simulink model "powerwindow"  (Simulink 7.9)
settings: Solver=ode45  StartTime=0.0  StopTime=inf  RelTol=1e-3
libraries: simulink x3
settings Model: Creator=ia3803  LastModifiedBy=ia3803

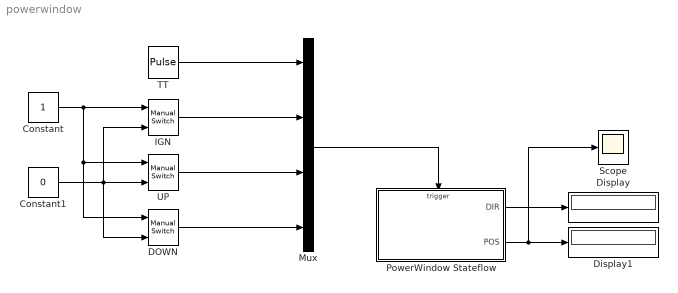
== system powerwindow ==
  Constant : Constant
  Constant1 : Constant  Value=0
  DOWN : simulink/Signal Routing/Manual Switch  sw=0  action=0  varsize=off
  Display : Display
  Display1 : Display
  IGN : simulink/Signal Routing/Manual Switch  sw=1  action=0  varsize=off
  Mux : Mux
  PowerWindow Stateflow : Stateflow chart  TreatAsAtomicUnit=on
  Scope : Scope
  TT : DiscretePulseGenerator  PulseType=Time based  Period=1  PulseWidth=50
  UP : simulink/Signal Routing/Manual Switch  sw=1  action=0  varsize=off
  wires:
  TT/1 -> Mux/1
  Constant/1 -> IGN/1, UP/1, DOWN/1
  Constant1/1 -> UP/2, DOWN/2, IGN/2
  IGN/1 -> Mux/2
  UP/1 -> Mux/3
  DOWN/1 -> Mux/4
  Mux/1 -> PowerWindow Stateflow/Trigger
  PowerWindow Stateflow/1(DIR) -> Display/1
  PowerWindow Stateflow/2(POS) -> Display1/1, Scope/1

== stateflow chart PowerWindow Stateflow ==
  state OFF
  state ON
    state STANDSTILL
      entry:
      DIR=0;
    state UP
      entry:
      DIR=2;
    state DOWN
      entry:
      DIR=1;
    DOWN -> STANDSTILL [order 2] : DOWN
    (default) -> STANDSTILL
    STANDSTILL -> UP [order 2] : UP[POS<20]
    UP -> STANDSTILL [order 1] : UP
    STANDSTILL -> DOWN [order 1] : DOWN[POS>0]
    UP -> STANDSTILL [order 2] : [POS==20]
    DOWN -> STANDSTILL [order 1] : [POS==0]
    DOWN -> DOWN [order 3] : TT[POS>0]/POS--;
    UP -> UP [order 3] : TT[POS<20]/POS++;
    DOWN -> UP [order 4] : UP
    UP -> DOWN [order 4] : DOWN
  OFF -> ON : IGN
  ON -> OFF : IGN
  (default) -> OFF : /DIR=0;POS=0;
  data: DIR output double; POS output double
  events: TT input EITHER_EDGE_EVENT; IGN input EITHER_EDGE_EVENT; UP input EITHER_EDGE_EVENT; DOWN input EITHER_EDGE_EVENT
